simulink model "verify_Absorption_Chiller_ddT_mdl"  (R2018b)
settings: Solver=ode45  StartTime=0  StopTime=3600  MaxStep=60  RelTol=1e-3  EnableMultiTasking=on
libraries: carnot x4
settings Model: Creator=drhf  LastModifiedBy=drhf
settings DataIOCC: SaveFormat=Array  SignalLoggingSaveFormat=ModelDataLogs
settings OptimizationCC: ExpressionDepthLimit=2147483647  LifeSpan=inf
settings DebuggingCC: UnderspecifiedInitializationDetection=Classic  MergeDetectMultiDrivingBlocksExec=none  SolverPrmCheckMsg=warning  FcnCallInpInsideContextMsg=warning  StateNameClashWarn=warning  SFUnexpectedBacktrackingDiag=warning  SFNoUnconditionalDefaultTransitionDiag=warning  SFExecutionAtInitializationDiag=none
settings HardwareCC: ProdBitPerPointer=32  ProdBitPerSizeT=32  ProdBitPerPtrDiffT=32  ProdLargestAtomicFloat=None  ProdIntDivRoundTo=Undefined  ProdEndianess=Unspecified  ProdWordSize=32  ProdHWDeviceType=32-bit Generic
settings ModelReferenceCC: PropagateSignalLabelsOutOfModel=off
settings SFSimCC: SimUseLocalCustomCode=off
settings RTWCC: RTWUseLocalCustomCode=off
settings CodeAppCC: StateflowObjectComments=on
settings GRTTargetCC: TargetLangStandard=C89/C90 (ANSI)  GeneratePreprocessorConditionals=Disable all  CombineOutputUpdateFcns=off  GRTInterface=on
settings ConfigComp: CovMetricSettings=dw  CovHtmlReporting=on  CovSaveCumulativeToWorkspaceVar=on  CovSaveSingleToWorkspaceVar=on  CovExternalEMLEnable=off

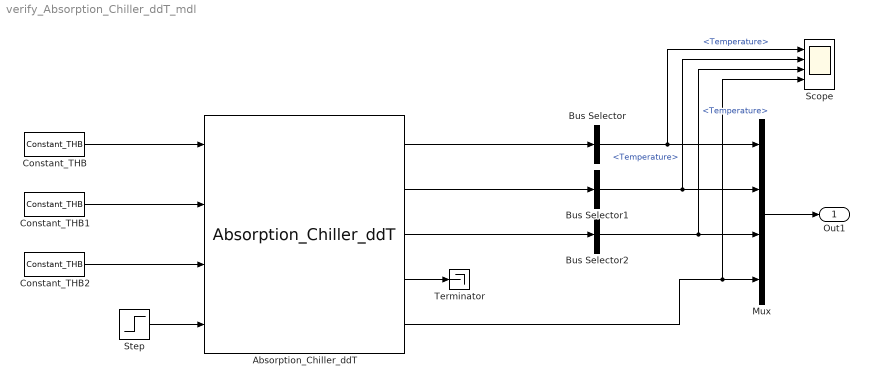
== system verify_Absorption_Chiller_ddT_mdl ==
  Absorption_Chiller_ddT : carnot/Source/Chiller/Absorption_Chiller_ddT  E=1.2  sE=0.42  rE=0.9  sG=0.51  rG=2/0.51  dpe=[100 1e4]  dpg=[100 1e4]  Pel_p=80
  Bus Selector : BusSelector  OutputSignals=Temperature
  Bus Selector1 : BusSelector  OutputSignals=Temperature
  Bus Selector2 : BusSelector  OutputSignals=Temperature
  Constant_THB : carnot/Source/Simple/Constant_THB  t=15  mdot=1200/3600  p=1e5  mID=No Pressure Drop  fluid=Water  mix=0  mix2=0  mix3=0  dia=0.02  hgt=0
  Constant_THB1 : carnot/Source/Simple/Constant_THB  t=90  mdot=1200/3600  p=1e5  mID=No Pressure Drop  fluid=Water  mix=0  mix2=0  mix3=0  dia=0.02  hgt=0
  Constant_THB2 : carnot/Source/Simple/Constant_THB  t=30  mdot=1200/3600  p=1e5  mID=No Pressure Drop  fluid=Water  mix=0  mix2=0  mix3=0  dia=0.02  hgt=0
  Mux : Mux
  Scope : Scope  NumInputPorts=4
  Step : Step  Time=0  SampleTime=0
  Terminator : Terminator
  Out1 : Outport
  wires:
  Mux/1 -> Out1/1
  Bus Selector/1 -> Mux/1, Scope/1  "<Temperature>"
  Constant_THB/1 -> Absorption_Chiller_ddT/1
  Step/1 -> Absorption_Chiller_ddT/4
  Constant_THB1/1 -> Absorption_Chiller_ddT/2
  Constant_THB2/1 -> Absorption_Chiller_ddT/3
  Absorption_Chiller_ddT/1 -> Bus Selector/1
  Absorption_Chiller_ddT/2 -> Bus Selector1/1
  Absorption_Chiller_ddT/3 -> Bus Selector2/1
  Absorption_Chiller_ddT/4 -> Terminator/1
  Bus Selector1/1 -> Mux/2, Scope/2  "<Temperature>"
  Bus Selector2/1 -> Mux/3, Scope/3  "<Temperature>"
  Absorption_Chiller_ddT/5 -> Mux/4, Scope/4
